simulink model "untitled1"  (R2018b)
settings: Solver=VariableStepAuto  StartTime=0.0  StopTime=10.0  RelTol=1e-3
values from neighbouring files (symbols this model uses):
  Tf = 0.015    [licentam18.m]
  Ts = Ts_crt_control    (= 3.33333333333e-05)    [licentam18.m]
libraries: simulink x1
settings Model: Creator=mocan  LastModifiedBy=mocan

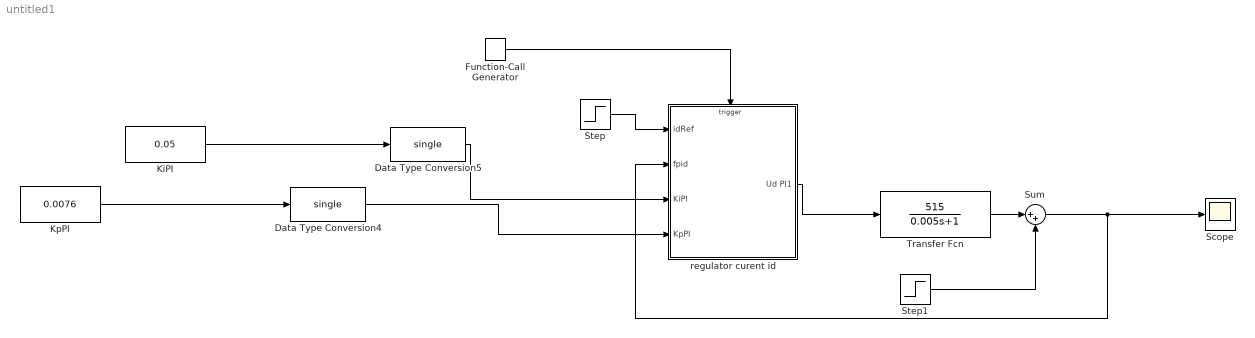
== system untitled1 ==
  Data Type Conversion4 : DataTypeConversion  OutDataTypeStr=single
  Data Type Conversion5 : DataTypeConversion  OutDataTypeStr=single
  Function-Call Generator : simulink/Ports & Subsystems/Function-Call Generator  sample_time=Ts_crt_control  numberOfIterations=1
  KiPI : Constant  Value=0.05
  KpPI : Constant  Value=0.0076
  Scope : Scope
  Step : Step  After=130  SampleTime=0
  Step1 : Step  Time=5  After=20  SampleTime=0
  Sum : Sum  Inputs=|++
  Transfer Fcn : TransferFcn  Numerator=[515]  Denominator=[0.005 1]
  regulator curent id : Subsystem
  wires:
  Data Type Conversion4/1 -> regulator curent id/4(KpPI)
  KiPI/1 -> Data Type Conversion5/1
  KpPI/1 -> Data Type Conversion4/1
  Data Type Conversion5/1 -> regulator curent id/3(KiPI)
  regulator curent id/1(Ud PI1) -> Transfer Fcn/1
  Step/1 -> regulator curent id/1(idRef)
  Function-Call Generator/1 -> regulator curent id/Trigger
  Step1/1 -> Sum/2
  Transfer Fcn/1 -> Sum/1
  Sum/1 -> regulator curent id/2(fpid), Scope/1

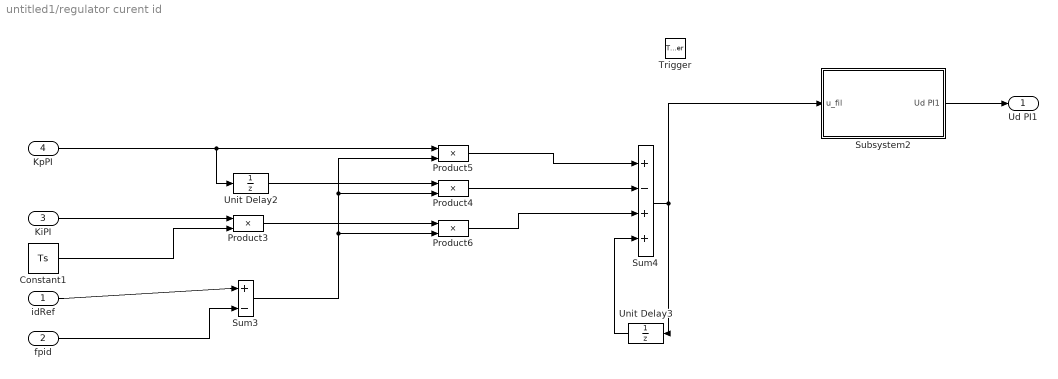
== system untitled1/regulator curent id ==
  idRef : Inport
  fpid : Inport  Port=2
  KiPI : Inport  Port=3
  KpPI : Inport  Port=4
  Trigger : TriggerPort  TriggerType=function-call  VariantControl=Variant  PortDimensions=1
  Constant1 : Constant  Value=Ts  OutDataTypeStr=single  SampleTime=-1
  Product{3..6} (4 alike) : Product
  Subsystem2 : Subsystem
  Sum3 : Sum  Inputs=|+-
  Sum4 : Sum  Inputs=+-++
  Unit Delay2 : UnitDelay  SampleTime=-1
  Unit Delay3 : UnitDelay  SampleTime=-1
  Ud PI1 : Outport
  wires:
  Product5/1 -> Sum4/1
  Product6/1 -> Sum4/3
  KpPI/1 -> Product5/1, Unit Delay2/1
  Unit Delay2/1 -> Product4/1
  Sum4/1 -> Subsystem2/1(u_fil), Unit Delay3/1
  Product4/1 -> Sum4/2
  Unit Delay3/1 -> Sum4/4
  Constant1/1 -> Product3/2
  idRef/1 -> Sum3/1
  KiPI/1 -> Product3/1
  fpid/1 -> Sum3/2
  Sum3/1 -> Product6/2, Product5/2, Product4/2
  Product3/1 -> Product6/1
  Subsystem2/1(Ud PI1) -> Ud PI1/1

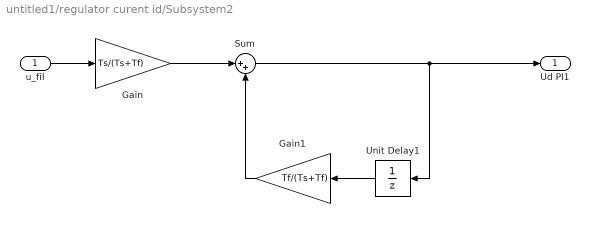
== system untitled1/regulator curent id/Subsystem2 ==
  u_fil : Inport
  Gain : Gain  Gain=Ts/(Ts+Tf)
  Gain1 : Gain  Gain=Tf/(Ts+Tf)
  Sum : Sum  Inputs=|++
  Unit Delay1 : UnitDelay  SampleTime=-1
  Ud PI1 : Outport
  wires:
  Sum/1 -> Ud PI1/1, Unit Delay1/1
  Gain/1 -> Sum/1
  Unit Delay1/1 -> Gain1/1
  u_fil/1 -> Gain/1
  Gain1/1 -> Sum/2
